simulink model "Der_Faux_FPGA_V2"  (R2020a)
settings: Solver=FixedStepDiscrete  StartTime=0.0  StopTime=0.84375  FixedStep=1/fs_sim  RelTol=1e-3
values from neighbouring files (symbols this model uses):
  ADC_res = 5    [Der_Faux_ctr_FPGA.m]
  ADC_res_G4 = 8    [Der_Faux_ctr_FPGA.m]
  C10 = 680e-12    (= 6.8e-10)    [Der_Faux_ctr_FPGA.m]
  C11 = 1e-9    (= 1e-09)    [Der_Faux_ctr_FPGA.m]
  C12 = 68e-9    (= 6.8e-08)    [Der_Faux_ctr_FPGA.m]
  C13 = 150e-9    (= 1.5e-07)    [Der_Faux_ctr_FPGA.m]
  C17 = 1e-6    (= 1e-06)    [Der_Faux_ctr_FPGA.m]
  C18 = 100e-9    (= 1e-07)    [Der_Faux_ctr_FPGA.m]
  C20 = 1e-6    (= 1e-06)    [Der_Faux_ctr_FPGA.m]
  C5 = 100e-12    (= 1e-10)    [Der_Faux_ctr_FPGA.m]
  C7 = 1e-6    (= 1e-06)    [Der_Faux_ctr_FPGA.m]
  D4_FL = D4_opt.FractionLength    [Der_Faux_ctr_FPGA.m]
  D4_opt = sfi(D4,len_D)    [Der_Faux_ctr_FPGA.m]
  D4_WL = D4_opt.WordLength    [Der_Faux_ctr_FPGA.m]
  D7_FL = D7_opt.FractionLength    [Der_Faux_ctr_FPGA.m]
  D7_opt = sfi(D7,len_D)    [Der_Faux_ctr_FPGA.m]
  D7_WL = D7_opt.WordLength    [Der_Faux_ctr_FPGA.m]
  D8_FL = D8_opt.FractionLength    [Der_Faux_ctr_FPGA.m]
  D8_opt = sfi(D8,len_D)    [Der_Faux_ctr_FPGA.m]
  D8_WL = D8_opt.WordLength    [Der_Faux_ctr_FPGA.m]
  Dcs1_FL = Dcs1_opt.FractionLength    [Der_Faux_ctr_FPGA.m]
  Dcs1_opt = sfi(Dcs1,len_D)    [Der_Faux_ctr_FPGA.m]
  Dcs1_WL = Dcs1_opt.WordLength    [Der_Faux_ctr_FPGA.m]
  Dcs2_FL = Dcs2_opt.FractionLength    [Der_Faux_ctr_FPGA.m]
  Dcs2_WL = Dcs2_opt.WordLength    [Der_Faux_ctr_FPGA.m]
  FP_frac = FP_len-10    (= 36)    [Der_Faux_ctr_FPGA.m]
  FP_len = 46    [Der_Faux_ctr_FPGA.m]
  fs = 48000    [Der_Faux_ctr_FPGA.m]
  fs_sim = fs*ovs    (= 6144000)    [Der_Faux_ctr_FPGA.m]
  G0 = 1/4.7e3    (= 0.000212765957447)    [Der_Faux_ctr_FPGA.m]
  G1 = 1/4.7e3    (= 0.000212765957447)    [Der_Faux_ctr_FPGA.m]
  G10 = 1/12e3    (= 8.33333333333e-05)    [Der_Faux_ctr_FPGA.m]
  G11 = 1/12e3    (= 8.33333333333e-05)    [Der_Faux_ctr_FPGA.m]
  G12 = 1/12e3    (= 8.33333333333e-05)    [Der_Faux_ctr_FPGA.m]
  G13 = 1/47e3    (= 2.12765957447e-05)    [Der_Faux_ctr_FPGA.m]
  G14 = 1/22e3    (= 4.54545454545e-05)    [Der_Faux_ctr_FPGA.m]
  G15 = 1/12e3    (= 8.33333333333e-05)    [Der_Faux_ctr_FPGA.m]
  G16 = 1/12e3    (= 8.33333333333e-05)    [Der_Faux_ctr_FPGA.m]
  G17 = 1/12e3    (= 8.33333333333e-05)    [Der_Faux_ctr_FPGA.m]
  G18 = 1/2.7e3    (= 0.00037037037037)    [Der_Faux_ctr_FPGA.m]
  G19 = 1/20e3    (= 5e-05)    [Der_Faux_ctr_FPGA.m]
  G20 = 1/10e3    (= 0.0001)    [Der_Faux_ctr_FPGA.m]
  G21 = 1/10e3    (= 0.0001)    [Der_Faux_ctr_FPGA.m]
  G5 = 1/22e3    (= 4.54545454545e-05)    [Der_Faux_ctr_FPGA.m]
  G7 = 1/12e3    (= 8.33333333333e-05)    [Der_Faux_ctr_FPGA.m]
  Gdem = 0.00096    [Der_Faux_ctr_FPGA.m]
  Gmod = 0.00096    [Der_Faux_ctr_FPGA.m]
  Gvar1_N = fi(Gvar1_N,0,ADC_res,0)    [Der_Faux_ctr_FPGA.m]
  Gvar2_N = fi(Gvar2_N,0,ADC_res,0)    [Der_Faux_ctr_FPGA.m]
  Gvar3_N = fi(Gvar3_N,0,ADC_res,0)    [Der_Faux_ctr_FPGA.m]
  Gvar4_N = fi(Gvar4_N,0,ADC_res_G4,0)    [Der_Faux_ctr_FPGA.m]
  input_space = linspace(0,2^ADC_res-1,2^ADC_res)    [Der_Faux_ctr_FPGA.m]
  input_space_G4 = linspace(0,2^ADC_res_G4-1,2^ADC_res_G4)    [Der_Faux_ctr_FPGA.m]
  input_spcae_extended = linspace(0,(2^ADC_res)^3-1,(2^ADC_res)^3)    [Der_Faux_ctr_FPGA.m]
  limit_Faux = 4.5    [Der_Faux_ctr_FPGA.m]
  limit_PT2399 = 2.5    [Der_Faux_ctr_FPGA.m]
  LUT_cd = fi(LUT_cd,0,LUT_cd_res,0)    [Der_Faux_ctr_FPGA.m]
  LUT_Gvar1_opt = sfi(LUT_Gvar1, len1)    [Der_Faux_ctr_FPGA.m]
  LUT_Gvar2_reversed_opt = sfi(LUT_Gvar2_reversed, len2)    [Der_Faux_ctr_FPGA.m]
  LUT_Gvar3_opt = sfi(LUT_Gvar3, len3)    [Der_Faux_ctr_FPGA.m]
  LUT_Z22a_opt = sfi(LUT_Z22a, len_LUT22a)    [Der_Faux_ctr_FPGA.m]
  LUT_Z22b_opt = sfi(LUT_Z22b, len_LUT22b)    [Der_Faux_ctr_FPGA.m]
  LUT_Z23a_opt = sfi(LUT_Z23a, len_Z23a)    [Der_Faux_ctr_FPGA.m]
  LUT_Z23b_opt = sfi(LUT_Z23b, len_Z23b)    [Der_Faux_ctr_FPGA.m]
  LUT_Z24a_opt = sfi(LUT_Z24a, len_LUT24a)    [Der_Faux_ctr_FPGA.m]
  LUT_Z24b_opt = sfi(LUT_Z24b, len_LUT24b)    [Der_Faux_ctr_FPGA.m]
  LUT_Z25a_opt = sfi(LUT_Z25a, len_LUT25a)    [Der_Faux_ctr_FPGA.m]
  LUT_Z25b_opt = sfi(LUT_Z25b, len_LUT25b)    [Der_Faux_ctr_FPGA.m]
  N4_FL = N4_opt.FractionLength    [Der_Faux_ctr_FPGA.m]
  N4_opt = sfi(N4,len_N)    [Der_Faux_ctr_FPGA.m]
  N4_WL = N4_opt.WordLength    [Der_Faux_ctr_FPGA.m]
  N7_FL = N7_opt.FractionLength    [Der_Faux_ctr_FPGA.m]
  N7_opt = sfi(N7,len_N)    [Der_Faux_ctr_FPGA.m]
  N7_WL = N7_opt.WordLength    [Der_Faux_ctr_FPGA.m]
  N8_FL = N8_opt.FractionLength    [Der_Faux_ctr_FPGA.m]
  N8_opt = sfi(N8,len_N)    [Der_Faux_ctr_FPGA.m]
  N8_WL = N8_opt.WordLength    [Der_Faux_ctr_FPGA.m]
  Ncs1_FL = Ncs1_opt.FractionLength    [Der_Faux_ctr_FPGA.m]
  Ncs1_opt = sfi(Ncs1,len_N)    [Der_Faux_ctr_FPGA.m]
  Ncs1_WL = Ncs1_opt.WordLength    [Der_Faux_ctr_FPGA.m]
  Ncs2_FL = Ncs2_opt.FractionLength    [Der_Faux_ctr_FPGA.m]
  Ncs2_WL = Ncs2_opt.WordLength    [Der_Faux_ctr_FPGA.m]
  shift_reg_size = 8*44000    (= 352000)    [Der_Faux_ctr_FPGA.m]
  use_stimuli = [true,true,true,true]    [Der_Faux_ctr_FPGA.m]
  w1 = 1e6    (= 1000000)    [Der_Faux_ctr_FPGA.m]
  w3 = 1e6    (= 1000000)    [Der_Faux_ctr_FPGA.m]
  w4 = 1e6    (= 1000000)    [Der_Faux_ctr_FPGA.m]
  w5 = 1e6    (= 1000000)    [Der_Faux_ctr_FPGA.m]
  w8 = 2*pi*3e6    (= 18849555.9215)    [Der_Faux_ctr_FPGA.m]
  WL_RAM = 5    [Der_Faux_ctr_FPGA.m]
undefined symbols (not defined in the file or in its folder): D10_FL, D10_opt, D10_WL, D11_FL, D11_opt, D11_WL, D13_FL, D13_opt, D13_WL, D16_FL, D16_opt, D16_WL, D20_FL, D20_opt, D20_WL, D21_FL, D21_opt, D21_WL, D26_FL, D26_opt, D26_WL, D27_FL, D27_opt, D27_WL, D28_FL, D28_opt, D28_WL, D29_FL, D29_opt, D29_WL, D30_FL, D30_opt, D30_WL, Dcs2, DiscIntNeverNeededParam, N10_FL, N10_opt, N10_WL, N11_FL, N11_opt, N11_WL, N13_FL, N13_opt, N13_WL, N16_FL, N16_opt, N16_WL, N20_FL, N20_opt, N20_WL, N21_FL, N21_opt, N21_WL, N26_FL, N26_opt, N26_WL, N27_FL, N27_opt, N27_WL, N28_FL ... (+13)
libraries: simulink x18, hdlsllib x4
(part 2 of 2)

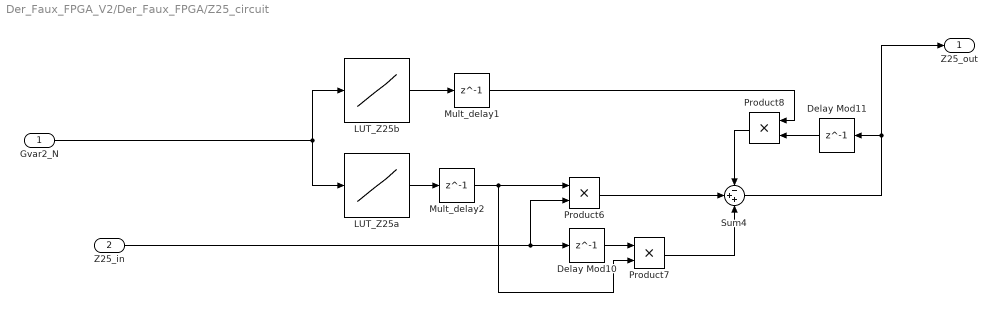
== system Der_Faux_FPGA_V2/Der_Faux_FPGA/Z25_circuit ==
  Gvar2_N : Inport  OutDataTypeStr=fixdt(0,ADC_res,0, 'DataTypeOverride', 'Off')  SampleTime=1/fs_sim  LockScale=on
  Z25_in : Inport  Port=2
  Delay Mod10 : Delay  DelayLength=1  InitialCondition=0  SampleTime=1/fs_sim
  Delay Mod11 : Delay  DelayLength=1  InitialCondition=0  SampleTime=1/fs_sim
  LUT_Z25a : Lookup_n-D  NumberOfTableDimensions=1  LookupTableObject=''  BreakpointsForDimension1=input_space  BreakpointsForDimension1FirstPoint=10  BreakpointsForDimension2FirstPoint=10  BreakpointsForDimension1Spacing=12  BreakpointsForDimension2Spacing=12  IndexSearchMethod=Evenly spaced points  Table=LUT_Z25a_opt  TableDataTypeStr=Inherit: Inherit from 'Table data'  InterpMethod=Flat  DiagnosticForOutOfRangeInput=Error  InternalRulePriority=Speed  OutDataTypeStr=Inherit: Inherit from 'Table data'  RndMeth=Simplest  InputSameDT=on  LockScale=on
  LUT_Z25b : Lookup_n-D  NumberOfTableDimensions=1  LookupTableObject=''  BreakpointsForDimension1=input_space  BreakpointsForDimension1FirstPoint=10  BreakpointsForDimension2FirstPoint=10  BreakpointsForDimension1Spacing=12  BreakpointsForDimension2Spacing=12  IndexSearchMethod=Evenly spaced points  Table=LUT_Z25b_opt  TableDataTypeStr=Inherit: Inherit from 'Table data'  InterpMethod=Flat  DiagnosticForOutOfRangeInput=Error  InternalRulePriority=Speed  OutDataTypeStr=Inherit: Inherit from 'Table data'  RndMeth=Simplest  InputSameDT=on  LockScale=on
  Mult_delay1 : Delay  DelayLength=1
  Mult_delay2 : Delay  DelayLength=1
  Product6 : Product  OutDataTypeStr=fixdt(1,FP_len, FP_frac)  SaturateOnIntegerOverflow=on
  Product7 : Product  OutDataTypeStr=fixdt(1,FP_len, FP_frac)  SaturateOnIntegerOverflow=on
  Product8 : Product  OutDataTypeStr=fixdt(1,FP_len, FP_frac)  SaturateOnIntegerOverflow=on
  Sum4 : Sum  Inputs=-++  OutDataTypeStr=fixdt(1,FP_len, FP_frac)  SaturateOnIntegerOverflow=on
  Z25_out : Outport
  wires:
  LUT_Z25b/1 -> Mult_delay1/1
  Gvar2_N/1 -> LUT_Z25b/1, LUT_Z25a/1
  Product8/1 -> Sum4/1
  Z25_in/1 -> Delay Mod10/1, Product6/2
  LUT_Z25a/1 -> Mult_delay2/1
  Product7/1 -> Sum4/3
  Delay Mod10/1 -> Product7/1
  Sum4/1 -> Z25_out/1, Delay Mod11/1
  Delay Mod11/1 -> Product8/2
  Product6/1 -> Sum4/2
  Mult_delay1/1 -> Product8/1
  Mult_delay2/1 -> Product7/2, Product6/1

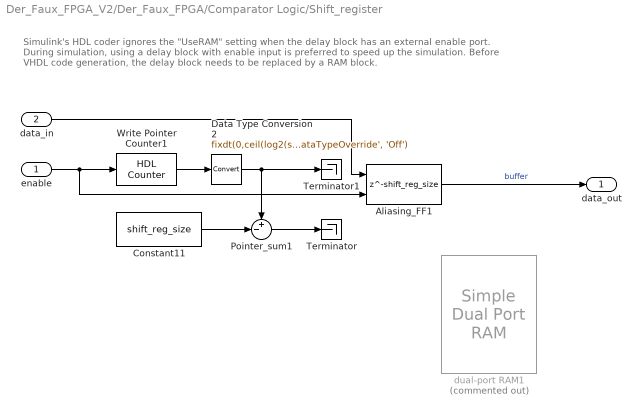
== system Der_Faux_FPGA_V2/Der_Faux_FPGA/Comparator Logic/Shift_register ==
  note: Simulink's HDL coder ignores the "UseRAM" setting when the delay block has an external enable port.
      | During simulation, using a delay block with enable input is preferred to speed up the simulation.
      | Before VHDL code generation, the delay block needs to be replaced by a RAM block.
  enable : Inport
  data_in : Inport  Port=2
  Aliasing_FF1 : Delay  DelayLength=shift_reg_size  InitialCondition=0  ShowEnablePort=on  SampleTime=1/(fs_sim)
      settings: InputPortMap=u0,e6
  Constant11 : Constant  Value=shift_reg_size  OutDataTypeStr=fixdt(0,ceil(log2(shift_reg_size)),0, 'DataTypeOverride', 'Off')  SampleTime=1/(fs_sim)  LockScale=on
  Data Type Conversion2 : DataTypeConversion  OutDataTypeStr=fixdt(0,ceil(log2(shift_reg_size)),0, 'DataTypeOverride', 'Off')  LockScale=on
  Pointer_sum1 : Sum  Inputs=+-|  OutDataTypeStr=fixdt(0,ceil(log2(shift_reg_size)),0, 'DataTypeOverride', 'Off')  LockScale=on
  Terminator : Terminator
  Terminator1 : Terminator
  Write Pointer Counter1 : hdlsllib/Sources/HDL Counter  CountType=Count limited  CountInit=0  CountStep=1  CountMax=2^ceil(log2(shift_reg_size))-1  CountFromType=Initial value  CountFrom=0  CountResetPort=off  CountLoadPort=off  CountEnbPort=on  CountDirPort=off  CountDataType=Unsigned  CountWordLen=ceil(log2(shift_reg_size))  CountFracLen=0  CountSampTime=1/(fs_sim/WL_RAM)
  dual-port RAM1 : hdlsllib/HDL RAMs/Simple Dual Port RAM  Commented=on  ram_size=ceil(log2(shift_reg_size))
      settings: SourceProductBaseCode=SL
  data_out : Outport
  wires:
  Aliasing_FF1/1 -> data_out/1  "buffer"
  Write Pointer Counter1/1 -> Data Type Conversion2/1
  data_in/1 -> Aliasing_FF1/1
  Pointer_sum1/1 -> Terminator/1
  Constant11/1 -> Pointer_sum1/2
  enable/1 -> Aliasing_FF1/2, Write Pointer Counter1/1
  Data Type Conversion2/1 -> Terminator1/1, Pointer_sum1/1
